simulink model "Demo_MinSegMotor_Nano33Iot_25a"  (R2025a)
settings: Solver=FixedStepDiscrete  StartTime=0.0  StopTime=inf  FixedStep=.005  RelTol=1e-3
libraries: arduinolib x7, arduinosensorlib x2
settings Model: SILPILModeSetting=veronly  ExtModeTrigDuration=2  Creator=Alec  LastModifiedBy=hurstj
settings SolverCC: AlgebraicLoopSolver=TrustRegion
settings DataIOCC: LimitDataPoints=on  SaveFormat=Array  SaveOutput=off  DSMLogging=off  SaveTime=off  ReturnWorkspaceOutputs=off
settings OptimizationCC: EnhancedBackFolding=on  PassReuseOutputArgsThreshold=0.0  ExpressionDepthLimit=2147483647.0  MaxStackSize=64  OptimizeBlockOrder=speed  DifferentSizesBufferReuse=on  OptimizationCustomize=off
settings DebuggingCC: UnderspecifiedInitializationDetection=Classic  MergeDetectMultiDrivingBlocksExec=none  ParameterTunabilityLossMsg=error  UnconnectedInputMsg=warning  UnconnectedOutputMsg=warning  UnconnectedLineMsg=warning  StateNameClashWarn=warning  SFUnexpectedBacktrackingDiag=warning  SFNoUnconditionalDefaultTransitionDiag=warning  SFExecutionAtInitializationDiag=none  ArithmeticOperatorsInVariantConditions=warning
settings HardwareCC: ProdBitPerPointer=32.0  ProdBitPerSizeT=32.0  ProdBitPerPtrDiffT=32.0  ProdLargestAtomicInteger=Long  ProdLargestAtomicFloat=Double  ProdWordSize=32.0  ProdHWDeviceType=ARM Compatible->ARM Cortex  UseEmbeddedCoderFeatures=off  UseSimulinkCoderFeatures=off
settings ModelReferenceCC: EnableRefExpFcnMdlSchedulingChecks=on  PropagateSignalLabelsOutOfModel=off
settings SFSimCC: SimUseLocalCustomCode=off  MATLABDynamicMemAlloc=off  CustomCodeUndefinedFunction=UseInterfaceOnly
settings RTWCC: SystemTargetFile=ert.tlc  HardwareBoard=Arduino Nano 33 IoT  TemplateMakefile=ert_default_tmf  RTWVerbose=off  RTWUseLocalCustomCode=off  Toolchain=Arduino ARM  BuildConfiguration=Faster Runs  GPUComputeCapability=3.5  DLArmComputeVersion=19.05  Description=Embedded Coder
settings CodeAppCC: ForceParamTrailComments=on  OperatorAnnotations=on  MangleLength=10.0
settings ERTTargetCC: ExtModeTransport=3.0  ExtModeAutomaticAllocSize=off  ExtModeStaticAllocSize=8192.0  InlinedParameterPlacement=Hierarchical  DynamicArrayContainerType=coder::array  ERTCustomFileBanners=off  SupportContinuousTime=on  SupportNonInlinedSFcns=on  RemoveResetFunc=off  SupportVariableSizeSignals=on  ModelStepFunctionPrototypeControlCompliant=off
settings ConfigComp: CovMetricSettings=dw  CovSaveCumulativeToWorkspaceVar=on  CovSaveSingleToWorkspaceVar=on  CovExternalEMLEnable=off

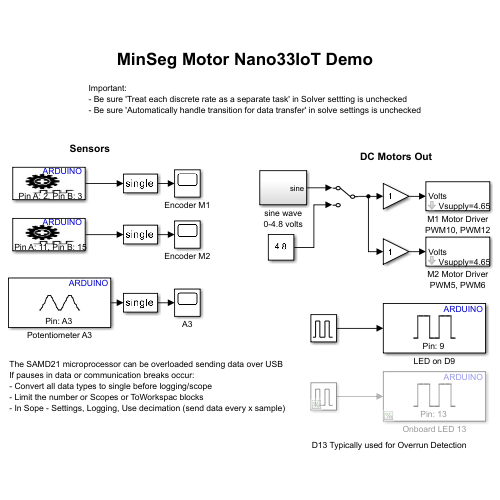
[thumbnail: Simulink's stored preview of the top-level diagram]
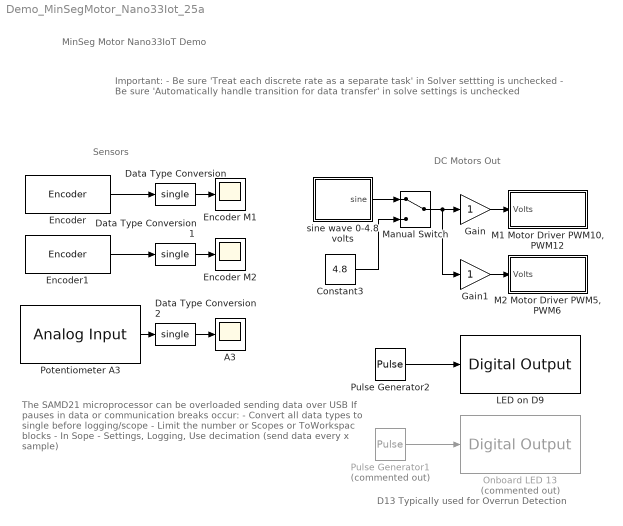
== system Demo_MinSegMotor_Nano33Iot_25a ==
  note: D13 Typically used for Overrun Detection
  note: DC Motors Out
  note: Sensors
  note: MinSeg Motor Nano33IoT Demo
  note: Important:
      | - Be sure 'Treat each discrete rate as a separate task' in Solver settting is unchecked
      | - Be sure 'Automatically handle transition for data transfer' in solve settings is unchecked
  note: The SAMD21 microprocessor can be overloaded sending data over USB
      | If pauses in data or communication breaks occur:
      | - Convert all data types to single before logging/scope
      | - Limit the number or Scopes or ToWorkspac blocks
      | - In Sope - Settings, Logging, Use decimation (send data every x sample)
  A3 : Scope
      settings: TimeSpan=30  ActiveDisplayYMinimum=-511.87499999999989  ActiveDisplayYMaximum=4606.875
  Constant3 : Constant  Value=4.8
  Data Type Conversion : DataTypeConversion  OutDataTypeStr=single  SaturateOnIntegerOverflow=off  RndMeth=Floor
  Data Type Conversion1 : DataTypeConversion  OutDataTypeStr=single  SaturateOnIntegerOverflow=off  RndMeth=Floor
  Data Type Conversion2 : DataTypeConversion  OutDataTypeStr=single  SaturateOnIntegerOverflow=off  RndMeth=Floor
  Encoder : arduinosensorlib/Encoder  InputA=2  InputB=3  Mode=No reset  SampleTime=-1
  Encoder M1 : Scope
      settings: TimeSpan=30  ActiveDisplayYMinimum=-9113.375  ActiveDisplayYMaximum=39720.375  DataLoggingVariableName=ScopeData2
  Encoder M2 : Scope
      settings: TimeSpan=30  ActiveDisplayYMinimum=-1  ActiveDisplayYMaximum=1
  Encoder1 : arduinosensorlib/Encoder  InputA=11  InputB=15  Mode=No reset  SampleTime=-1
  Gain : Gain
  Gain1 : Gain
  LED on D9 : arduinolib/Digital Output  pinNumber=9  Direction=output  blockPlatform=arduino
  "M1 Motor Driver PWM10, PWM12" : Subsystem  mask{Vsupply=4.65, Voffset=0}
      mask prompts: Vsupply "Driver Voltage"
      mask help:
      | Specify driver supply voltage (around 4.9 for USB, 8.7 for 6AA batteries)
      | Specify the Voltage offset (0-Vsupply)
      |
      | Driver supply voltage can be measured direcly by turning the motor fully on (100% duty cycle) and measuring the voltage across the motor leads.  This is the maximum voltage available to the motor and is used to scale from volts to PWM value 0-255.
      |
      | Note this value must be changed if the supply voltage to the driver is changed, for example, by using batteries.
      |
      | Vsupply is the maximum voltage your system is capable of supplying to system given the power supply. It needs to be measured depending on the power supply.
      mask Display:
      | port_label('input',1,'Volts')
      | text(15,5,['Vsupply=' num2str(Vsupply)])
  "M2 Motor Driver PWM5, PWM6" : Subsystem  mask{Vsupply=4.65, Voffset=0}
      mask prompts: Vsupply "Driver Voltage"
      mask help:
      | Specify driver supply voltage (around 4.9 for USB, 8.7 for 6AA batteries)
      | Specify the Voltage offset (0-Vsupply)
      |
      | Driver supply voltage can be measured direcly by turning the motor fully on (100% duty cycle) and measuring the voltage across the motor leads.  This is the maximum voltage available to the motor and is used to scale from volts to PWM value 0-255.
      |
      | Note this value must be changed if the supply voltage to the driver is changed, for example, by using batteries.
      |
      | Vsupply is the maximum voltage your system is capable of supplying to system given the power supply. It needs to be measured depending on the power supply.
      mask Display:
      | port_label('input',1,'Volts')
      | text(15,5,['Vsupply=' num2str(Vsupply)])
  Manual Switch : ManualSwitch
  Onboard LED 13 : arduinolib/Digital Output  Commented=on  pinNumber=13  Direction=output  blockPlatform=arduino
  Potentiometer A3 : arduinolib/Analog Input  pinNumber=3  ReadResultsOnly=off  ConversionTriggerSource=Software  ExternalTriggerType=uint32( 0 )  OutputDataType=uint16  EnableConversionCompleteNotify=off  EnableOuputStatus=off  SampleTime=-1  blockPlatform=arduino
  Pulse Generator1 : DiscretePulseGenerator  Commented=on  PulseType=Time based  Period=1  PulseWidth=50
  Pulse Generator2 : DiscretePulseGenerator  PulseType=Time based  Period=1  PulseWidth=50
  sine wave 0-4.8 volts : Subsystem
  wires:
  Pulse Generator1/1 -> Onboard LED 13/1
  Gain/1 -> "M1 Motor Driver PWM10, PWM12"/1(Volts)
  Gain1/1 -> "M2 Motor Driver PWM5, PWM6"/1(Volts)
  Encoder1/1 -> Data Type Conversion1/1
  Encoder/1 -> Data Type Conversion/1
  Manual Switch/1 -> Gain1/1, Gain/1
  sine wave 0-4.8 volts/1(sine) -> Manual Switch/1
  Constant3/1 -> Manual Switch/2
  Pulse Generator2/1 -> LED on D9/1
  Data Type Conversion/1 -> Encoder M1/1
  Data Type Conversion1/1 -> Encoder M2/1
  Potentiometer A3/1 -> Data Type Conversion2/1
  Data Type Conversion2/1 -> A3/1

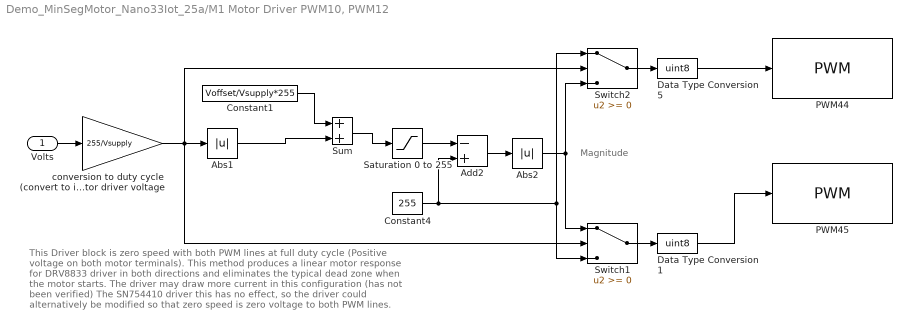
== system Demo_MinSegMotor_Nano33Iot_25a/M1 Motor Driver PWM10, PWM12 ==
  note: This Driver block is zero speed with both PWM lines at full duty cycle
      |  (Positive voltage on both motor terminals).
      | This method produces a linear motor response for DRV8833 driver
      |  in both directions and eliminates
      | the typical dead zone when the motor starts.
      | The driver may draw more current in this configuration (has not been verified)
      |
      | The SN754410 driver this has no effect, so the driver could alternatively
      | be modified so that zero speed is zero voltage to both PWM lines.
  note: Magnitude
  Volts : Inport
  Abs1 : Abs  SaturateOnIntegerOverflow=off
  Abs2 : Abs  SaturateOnIntegerOverflow=off
  Add2 : Sum  Inputs=-+
  Constant1 : Constant  Value=Voffset/Vsupply*255
  Constant4 : Constant  Value=255
  Data Type Conversion1 : DataTypeConversion  OutDataTypeStr=uint8  SaturateOnIntegerOverflow=off  RndMeth=Floor
  Data Type Conversion5 : DataTypeConversion  OutDataTypeStr=uint8  SaturateOnIntegerOverflow=off  RndMeth=Floor
  PWM44 : arduinolib/PWM  pinNumber=10  frequencyType=Specify  desiredFrequency=4000  achievableFrequency=4000
  PWM45 : arduinolib/PWM  pinNumber=12  frequencyType=Specify  desiredFrequency=4000  achievableFrequency=3989.3617
  Saturation 0 to 255 : Saturate  UpperLimit=255  LowerLimit=0
  Sum : Sum
  Switch1 : Switch  SaturateOnIntegerOverflow=off  InputSameDT=off
  Switch2 : Switch  SaturateOnIntegerOverflow=off  InputSameDT=off
  conversion to duty cycle (convert to int) denominator is motor driver voltage : Gain  Gain=255/Vsupply  OutDataTypeStr=int16
  wires:
  Abs1/1 -> Sum/2
  Sum/1 -> Saturation 0 to 255/1
  Constant1/1 -> Sum/1
  Volts/1 -> conversion to duty cycle (convert to int) denominator is motor driver voltage/1
  conversion to duty cycle (convert to int) denominator is motor driver voltage/1 -> Switch2/2, Abs1/1, Switch1/2
  Saturation 0 to 255/1 -> Add2/1
  Constant4/1 -> Switch1/3, Switch2/1, Add2/2
  Add2/1 -> Abs2/1
  Abs2/1 -> Switch2/3, Switch1/1
  Switch2/1 -> Data Type Conversion5/1
  Switch1/1 -> Data Type Conversion1/1
  Data Type Conversion5/1 -> PWM44/1
  Data Type Conversion1/1 -> PWM45/1

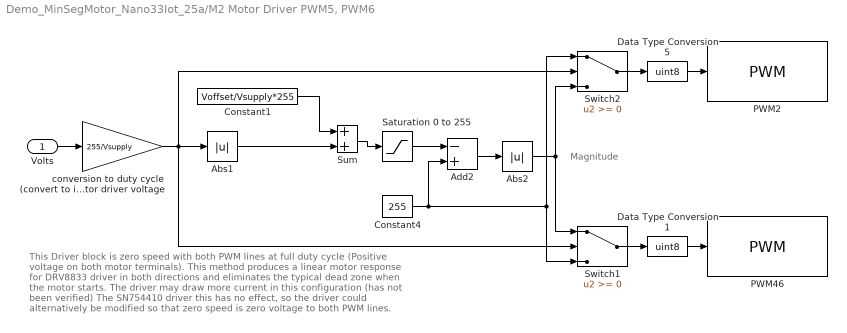
== system Demo_MinSegMotor_Nano33Iot_25a/M2 Motor Driver PWM5, PWM6 ==
  note: This Driver block is zero speed with both PWM lines at full duty cycle
      |  (Positive voltage on both motor terminals).
      | This method produces a linear motor response for DRV8833 driver
      |  in both directions and eliminates
      | the typical dead zone when the motor starts.
      | The driver may draw more current in this configuration (has not been verified)
      |
      | The SN754410 driver this has no effect, so the driver could alternatively
      | be modified so that zero speed is zero voltage to both PWM lines.
  note: Magnitude
  Volts : Inport
  Abs1 : Abs  SaturateOnIntegerOverflow=off
  Abs2 : Abs  SaturateOnIntegerOverflow=off
  Add2 : Sum  Inputs=-+
  Constant1 : Constant  Value=Voffset/Vsupply*255
  Constant4 : Constant  Value=255
  Data Type Conversion1 : DataTypeConversion  OutDataTypeStr=uint8  SaturateOnIntegerOverflow=off  RndMeth=Floor
  Data Type Conversion5 : DataTypeConversion  OutDataTypeStr=uint8  SaturateOnIntegerOverflow=off  RndMeth=Floor
  PWM2 : arduinolib/PWM  pinNumber=5  frequencyType=Specify  desiredFrequency=4000  achievableFrequency=4000
  PWM46 : arduinolib/PWM  pinNumber=6  frequencyType=Specify  desiredFrequency=4000  achievableFrequency=4000
  Saturation 0 to 255 : Saturate  UpperLimit=255  LowerLimit=0
  Sum : Sum
  Switch1 : Switch  SaturateOnIntegerOverflow=off  InputSameDT=off
  Switch2 : Switch  SaturateOnIntegerOverflow=off  InputSameDT=off
  conversion to duty cycle (convert to int) denominator is motor driver voltage : Gain  Gain=255/Vsupply  OutDataTypeStr=int16
  wires:
  Abs1/1 -> Sum/2
  Sum/1 -> Saturation 0 to 255/1
  Constant1/1 -> Sum/1
  Volts/1 -> conversion to duty cycle (convert to int) denominator is motor driver voltage/1
  conversion to duty cycle (convert to int) denominator is motor driver voltage/1 -> Abs1/1, Switch2/2, Switch1/2
  Saturation 0 to 255/1 -> Add2/1
  Constant4/1 -> Switch1/3, Switch2/1, Add2/2
  Add2/1 -> Abs2/1
  Abs2/1 -> Switch2/3, Switch1/1
  Switch2/1 -> Data Type Conversion5/1
  Switch1/1 -> Data Type Conversion1/1
  Data Type Conversion5/1 -> PWM2/1
  Data Type Conversion1/1 -> PWM46/1

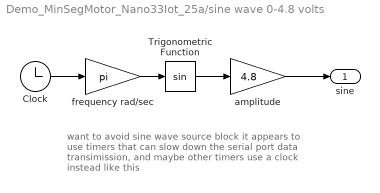
== system Demo_MinSegMotor_Nano33Iot_25a/sine wave 0-4.8 volts ==
  note: want to avoid sine wave source block
      | it appears to use timers that can slow down the
      | serial port data transimission, and maybe
      | other timers
      |
      | use a clock instead like this
  Clock : Clock
  Trigonometric Function : Trigonometry
  amplitude : Gain  Gain=4.8
  frequency rad/sec : Gain  Gain=pi
  sine : Outport
  wires:
  amplitude/1 -> sine/1
  frequency rad/sec/1 -> Trigonometric Function/1
  Trigonometric Function/1 -> amplitude/1
  Clock/1 -> frequency rad/sec/1
